simulink model "Signalflussplan2"  (R2026a)
settings: Solver=VariableStepAuto  StopTime=1.0
values from neighbouring files (symbols this model uses):
  b1 = 2.39e6    (= 2390000)    [variablen.m]    (also in variablen2.m; variablen4.m)
  c_o = 36.5e6    (= 36500000)    [variablen.m]    (also in variablen2.m; variablen4.m)
  c_p = 75e6    (= 75000000)    [variablen.m]    (also in variablen2.m; variablen4.m)
  FN = F_N    (= 63000)    [variablen.m]    (also in variablen2.m; variablen4.m)
  i_vmax = 1    [variablen.m]    (also in variablen2.m; variablen4.m)
  K_L = 1    [variablen.m]    (also in variablen2.m; variablen4.m)
  K_sv = 0.796    [variablen.m]    (also in variablen2.m; variablen4.m)
  m_g = m_k + m_p    (= 268.7)    [variablen.m]    (also in variablen2.m; variablen4.m)
settings Model: Creator=johannakruger
settings DataIOCC: ExternalInput=[0 0]  InitialState=[]  LoadInitialState=on
settings OptimizationCC: BufferReuse=off
settings DebuggingCC: InitInArrayFormatMsg=none

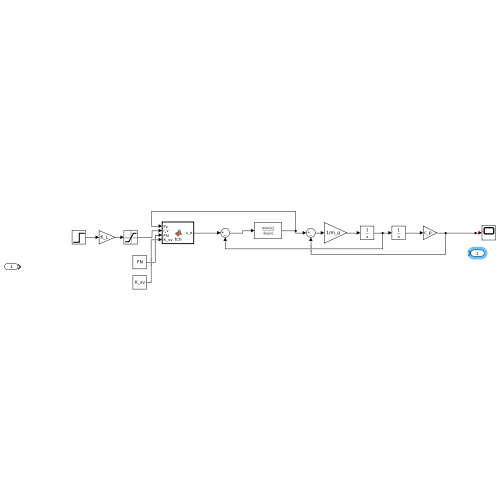
[thumbnail: Simulink's stored preview of the top-level diagram]
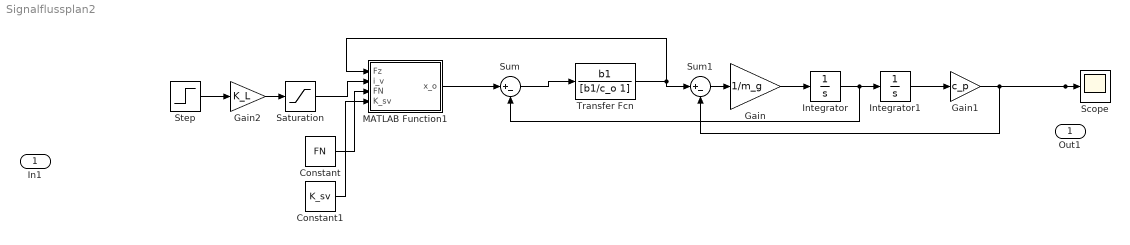
== system Signalflussplan2 ==
  In1 : Inport
  Constant : Constant  Value=FN
  Constant1 : Constant  Value=K_sv
  Gain : Gain  Gain=1/m_g
  Gain1 : Gain  Gain=c_p
  Gain2 : Gain  Gain=K_L
  Integrator : Integrator
  Integrator1 : Integrator
  MATLAB Function1 : MATLAB Function  TreatAsAtomicUnit=on
  Saturation : Saturate  UpperLimit=i_vmax  LowerLimit=-i_vmax
  Scope : Scope
      settings: ActiveDisplayYMinimum=-0.91190357323111926  ActiveDisplayYMaximum=0.902155383684981
  Step : Step  SampleTime=0
  Sum : Sum  Inputs=|+-
  Sum1 : Sum  Inputs=|+-
  Transfer Fcn : TransferFcn  Numerator=b1  Denominator=[b1/c_o 1]
  Out1 : Outport
  wires:
  Saturation/1 -> MATLAB Function1/2(i_v)
  Gain/1 -> Integrator/1
  Integrator1/1 -> Gain1/1
  MATLAB Function1/1(x_o) -> Sum/1
  Sum/1 -> Transfer Fcn/1
  Integrator/1 -> Sum/2, Integrator1/1
  Sum1/1 -> Gain/1
  Gain1/1 -> Sum1/2, Scope/1
  Transfer Fcn/1 -> Sum1/1, MATLAB Function1/1(Fz)
  Constant/1 -> MATLAB Function1/3(FN)
  Constant1/1 -> MATLAB Function1/4(K_sv)
  Gain2/1 -> Saturation/1
  Step/1 -> Gain2/1

== matlab function Signalflussplan2/MATLAB Function1 ==
  data: Fz input; i_v input; x_o output; FN input; K_sv input
function x_o = fcn(Fz, i_v, FN, K_sv)

A = 1 - Fz/FN * sign(i_v);

if A <= 0
    x_o = 0;
else
    x_o = i_v * K_sv * sqrt(A);
end
